simulink model "sumlationlab12"  (R2017a)
settings: Solver=VariableStepAuto  StartTime=0.0  StopTime=2  RelTol=1e-3
values from neighbouring files (symbols this model uses):
  D2 = Fs*0.25    (= 11025)    [lab12.m]    (also in lab_12.m)
  Fs = 250    [PS_Lab9_p3.m]    (also in lab12.m = 44100; lab_12.m = 44100)
settings Model: Creator=gerar  LastModifiedBy=gerar

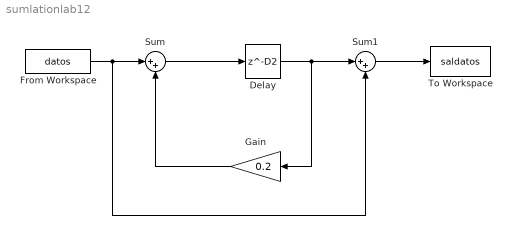
== system sumlationlab12 ==
  Delay : Delay  DelayLength=D2  InitialCondition=0
  From Workspace : FromWorkspace  VariableName=datos  SampleTime=1/Fs  OutputAfterFinalValue=Setting to zero
  Gain : Gain  Gain=0.2
  Sum : Sum  Inputs=|++
  Sum1 : Sum  Inputs=|++
  To Workspace : ToWorkspace  VariableName=saldatos  SampleTime=-1
  wires:
  Gain/1 -> Sum/2
  Sum/1 -> Delay/1
  Delay/1 -> Gain/1, Sum1/1
  From Workspace/1 -> Sum1/2, Sum/1
  Sum1/1 -> To Workspace/1
